simulink model "sldvdemo_debounce_adapted"  (R2017b)
settings: Solver=FixedStepDiscrete  StartTime=0.0  StopTime=10.0  FixedStep=0.01  RelTol=1e-3  EnableMultiTasking=on
undefined symbols (not defined in the file): sldvsubsys
libraries: sldvdemowidgets x2, sldvlib x1
Description:
  | Property Proving with an Assumption Block
  | 
  | This example shows how to perform a Simulink Design Verifier property proof using a
  | Proof Assumption block.
settings Model: Creator=The MathWorks, Inc.  LastModifiedBy=hbourbou
settings SolverCC: InsertRTBMode=Auto
settings DataIOCC: LimitDataPoints=on  SaveFormat=Array
settings OptimizationCC: DefaultParameterBehavior=Inlined  ExpressionDepthLimit=2147483647  InitFltsAndDblsToZero=on  EfficientMapNaN2IntZero=off  LifeSpan=inf
settings DebuggingCC: SaveWithParameterizedLinksMsg=none  UnderspecifiedInitializationDetection=Classic  MergeDetectMultiDrivingBlocksExec=none  SignalResolutionControl=TryResolveAllWithWarning  SolverPrmCheckMsg=warning  FcnCallInpInsideContextMsg=warning  StateNameClashWarn=warning  StrictBusMsg=Warning  SFUnexpectedBacktrackingDiag=warning  SFNoUnconditionalDefaultTransitionDiag=warning  SFExecutionAtInitializationDiag=none
settings HardwareCC: ProdBitPerPointer=32  ProdBitPerSizeT=32  ProdBitPerPtrDiffT=32  ProdLargestAtomicFloat=None  ProdIntDivRoundTo=Undefined  ProdEndianess=Unspecified  ProdWordSize=32  ProdHWDeviceType=32-bit Generic
settings ModelReferenceCC: PropagateSignalLabelsOutOfModel=off
settings SFSimCC: SimParseCustomCode=off
settings CodeAppCC: StateflowObjectComments=on
settings GRTTargetCC: TargetFcnLib=ansi_tfl_tmw.mat  TargetLangStandard=C89/C90 (ANSI)  GeneratePreprocessorConditionals=Disable all  CombineOutputUpdateFcns=off  GRTInterface=on
settings ConfigComp: DVMode=PropertyProving  DVMaxProcessTime=1200  DVMakeOutputFilesUnique=off  DVParameters=on  DVModelCoverageObjectives=MCDC  DVMaxTestCaseSteps=500  DVTestSuiteOptimization=CombinedObjectives  DVAssertions=EnableAll  DVProofAssumptions=EnableAll  DVDetectActiveLogic=on  DVDetectFloatOverflow=off  DVModelReferenceHarness=on

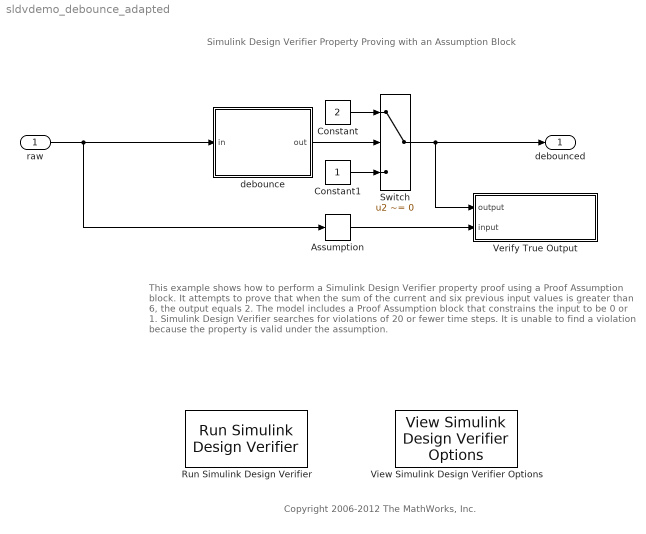
== system sldvdemo_debounce_adapted ==
  note: Copyright 2006-2012 The MathWorks, Inc.
  note: This example shows how to perform a Simulink Design Verifier property proof using a
      | Proof Assumption block. It attempts to prove that when the sum of the current and six
      | previous input values is greater than 6, the output equals 2. The model includes a
      | Proof Assumption block that constrains the input to be 0 or 1.
      |
      | Simulink Design Verifier searches for violations of 20 or fewer time steps.  It is unable
      | to find a violation because the property is valid under the assumption.
  note: Simulink Design Verifier
      | Property Proving with an Assumption Block
  raw : Inport  OutDataTypeStr=double
  Assumption : sldvlib/Objectives and Constraints/Assumption  enabled=on  customAVTBlockType=Assumption  intervals={0, 1}  initial=off  dispValues=on  outEnabled=on
      settings: AttributesFormatString=%<intervals>  SourceProductName=Simulink Design Verifier  SourceProductBaseCode=DV
  Constant : Constant  Value=2  OutDataTypeStr=uint8
  Constant1 : Constant  OutDataTypeStr=uint8
  "Run Simulink Design Verifier " : sldvdemowidgets/Run Simulink Design Verifier   SystemSampleTime=-1
      settings: SourceProductName=Simulink Design Verifier  SourceProductBaseCode=DV
  Switch : Switch  Criteria=u2 ~= 0
  Verify True Output : Subsystem  Tag=VerificationSubsystem  DisableCoverage=on  LoadFcn=sldvsubsys('check')  TreatAsAtomicUnit=on  SimViewingDevice=on  mask(VerificationSubsystem){}
      mask init:
      | sldvsubsys('maskInit');
      settings: CopyFcn=sldvsubsys('copy');
      settings: PreSaveFcn=|
      | set_param(gcb,'SimViewingDevice','on');
      | sldvsubsys('check');
      mask Display: image(imread('sldvicon_versubsys.png','BackGroundColor',[1 1 1]),'center');
  View Simulink Design Verifier Options : sldvdemowidgets/View Simulink Design Verifier Options  SystemSampleTime=-1
      settings: SourceProductName=Simulink Design Verifier  SourceProductBaseCode=DV
  debounce : Stateflow chart  TreatAsAtomicUnit=on
  debounced : Outport  OutDataTypeStr=uint8
  wires:
  debounce/1(out) -> Switch/2
  Switch/1 -> debounced/1, Verify True Output/1(output)
  Constant/1 -> Switch/1
  Constant1/1 -> Switch/3
  Assumption/1 -> Verify True Output/2(input)
  raw/1 -> Assumption/1, debounce/1(in)

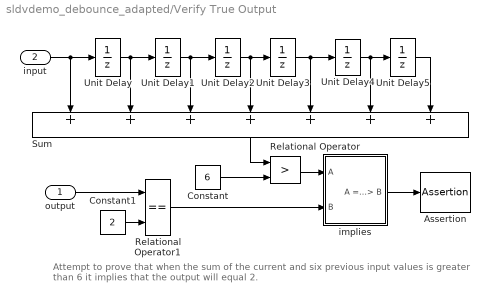
== system sldvdemo_debounce_adapted/Verify True Output ==
  note: Attempt to prove that when the sum of the current and six previous input
      | values is greater than 6 it implies that the output will equal 2.
  output : Inport
  input : Inport  Port=2
  Assertion : Assertion
  Constant : Constant  Value=6  OutDataTypeStr=double
  Constant1 : Constant  Value=2  OutDataTypeStr=uint8
  Relational Operator : RelationalOperator  Operator=>  OutDataTypeStr=boolean  RndMeth=Nearest
  Relational Operator1 : RelationalOperator  Operator===  OutDataTypeStr=boolean  RndMeth=Nearest
  Sum : Sum  Inputs=+++++++
  Unit Delay{,1..5} (6 alike) : UnitDelay  SampleTime=-1
  implies : Subsystem
  wires:
  input/1 -> Unit Delay/1, Sum/1
  Unit Delay/1 -> Unit Delay1/1, Sum/2
  Unit Delay1/1 -> Unit Delay2/1, Sum/3
  Unit Delay2/1 -> Unit Delay3/1, Sum/4
  Unit Delay3/1 -> Unit Delay4/1, Sum/5
  Unit Delay4/1 -> Sum/6, Unit Delay5/1
  Sum/1 -> Relational Operator/1
  Constant/1 -> Relational Operator/2
  Constant1/1 -> Relational Operator1/2
  output/1 -> Relational Operator1/1
  Relational Operator/1 -> implies/1(A)
  Relational Operator1/1 -> implies/2(B)
  implies/1(A ==> B) -> Assertion/1
  Unit Delay5/1 -> Sum/7

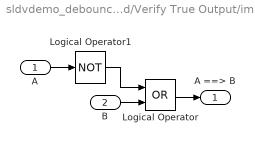
== system sldvdemo_debounce_adapted/Verify True Output/implies ==
  A : Inport
  B : Inport  Port=2
  Logical Operator : Logic  Operator=OR  AllPortsSameDT=off  OutDataTypeStr=boolean
  Logical Operator1 : Logic  Operator=NOT  AllPortsSameDT=off  OutDataTypeStr=boolean
  A ==> B : Outport
  wires:
  Logical Operator1/1 -> Logical Operator/1
  A/1 -> Logical Operator1/1
  Logical Operator/1 -> A ==> B/1
  B/1 -> Logical Operator/2

== stateflow chart sldvdemo_debounce_adapted/debounce ==
  settings: updateMethod=DISCRETE  sampleTime=0.01
  state To_on
    en: cnt = 0.0;
    du: cnt = cnt + 1;
  state Off
    en: out = false;
  state To_off
    en: cnt = 0.0;
    du: cnt = cnt + 1;
  state On
    en: out = true;
  (default) -> Off
  Off -> To_on : [in==1.0]
  To_on -> Off [order 1] : [in==0.0]
  To_off -> Off [order 2] : [cnt == 4.0]
  To_on -> On [order 2] : [cnt == 4.0]
  On -> To_off : [in==0.0]
  To_off -> On [order 1] : [in==1.0]
  data: in input double; out output boolean; cnt local double
